simulink library "Propulsion"  (R2024a)
settings: Solver=VariableStepAuto  StartTime=0.0  StopTime=10.0  RelTol=1e-3
undefined symbols (not defined in the file): Alpha_F, nrho, nv, rho_ref, T_max, use_linear_thrust, V_ref, X_F, Z_F
settings Model: Creator=mahariansyah  LastModifiedBy=mahariansyah

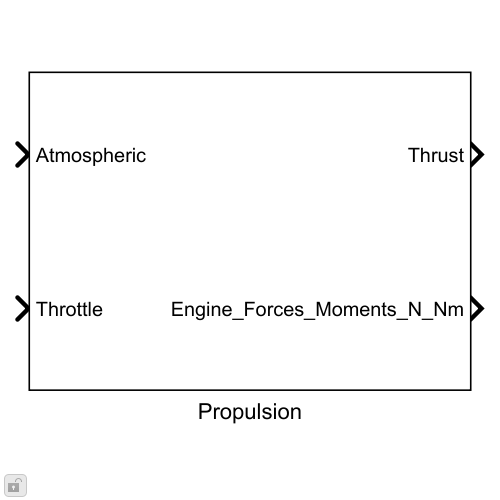
[thumbnail: Simulink's stored preview of the top-level diagram]
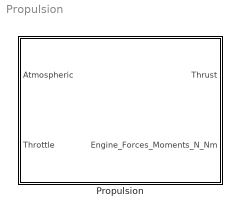
== system Propulsion ==
  Propulsion : Subsystem

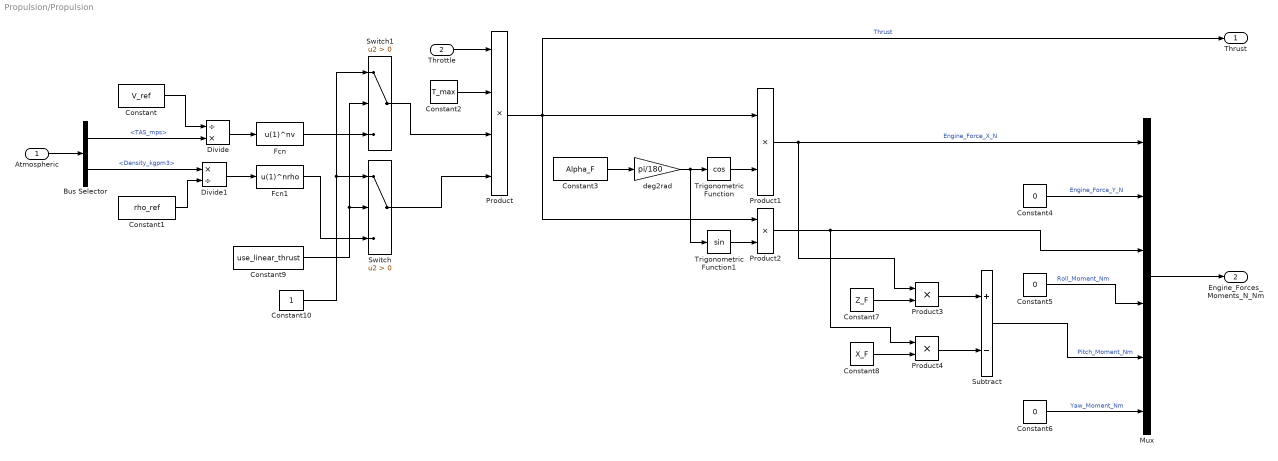
== system Propulsion/Propulsion ==
  Atmospheric : Inport
  Throttle : Inport  Port=2
  Bus Selector : BusSelector  OutputSignals=TAS_mps,Density_kgpm3
  Constant : Constant  Value=V_ref
  Constant1 : Constant  Value=rho_ref
  Constant10 : Constant
  Constant2 : Constant  Value=T_max
  Constant3 : Constant  Value=Alpha_F
  Constant4 : Constant  Value=0
  Constant5 : Constant  Value=0
  Constant6 : Constant  Value=0
  Constant7 : Constant  Value=Z_F
  Constant8 : Constant  Value=X_F
  Constant9 : Constant  Value=use_linear_thrust
  Divide : Product  Inputs=/*
  Divide1 : Product  Inputs=*/
  Fcn : Fcn  Expr=u(1)^nv
  Fcn1 : Fcn  Expr=u(1)^nrho
  Mux : Mux  Inputs=6
  Product : Product  Inputs=4
  Product{1..4} (4 alike) : Product
  Subtract : Sum  Inputs=+-
  Switch : Switch  Criteria=u2 > Threshold  SaturateOnIntegerOverflow=off  InputSameDT=off
  Switch1 : Switch  Criteria=u2 > Threshold  SaturateOnIntegerOverflow=off  InputSameDT=off
  Trigonometric Function : Trigonometry  Operator=cos
  Trigonometric Function1 : Trigonometry
  deg2rad : Gain  Gain=pi/180
  Thrust : Outport
  Engine_Forces_Moments_N_Nm : Outport  Port=2
  wires:
  Bus Selector/2 -> Divide1/1  "<Density_kgpm3>"
  Bus Selector/1 -> Divide/2  "<TAS_mps>"
  Product2/1 -> Mux/3, Product4/1
  Subtract/1 -> Mux/5  "Pitch_Moment_Nm"
  Constant4/1 -> Mux/2  "Engine_Force_Y_N"
  Constant5/1 -> Mux/4  "Roll_Moment_Nm"
  Constant6/1 -> Mux/6  "Yaw_Moment_Nm"
  Atmospheric/1 -> Bus Selector/1
  Constant1/1 -> Divide1/2
  Mux/1 -> Engine_Forces_Moments_N_Nm/1
  Constant8/1 -> Product4/2
  Product4/1 -> Subtract/2
  Product1/1 -> Product3/1, Mux/1  "Engine_Force_X_N"
  Product/1 -> Thrust/1, Product2/1, Product1/1  "Thrust"
  Constant7/1 -> Product3/2
  Product3/1 -> Subtract/1
  Throttle/1 -> Product/1
  Trigonometric Function1/1 -> Product2/2
  Constant/1 -> Divide/1
  Constant3/1 -> deg2rad/1
  Divide/1 -> Fcn/1
  Divide1/1 -> Fcn1/1
  deg2rad/1 -> Trigonometric Function1/1, Trigonometric Function/1
  Trigonometric Function/1 -> Product1/2
  Constant2/1 -> Product/2
  Switch/1 -> Product/4
  Switch1/1 -> Product/3
  Constant10/1 -> Switch1/1, Switch/1
  Fcn/1 -> Switch1/3
  Fcn1/1 -> Switch/3
  Constant9/1 -> Switch/2, Switch1/2
